simulink model "UnderwaterGliderLongModel2021b"  (R2021b)
settings: Solver=VariableStepAuto  StartTime=0.0  StopTime=inf  FixedStep=0.0000111111111111111111111111111  RelTol=1e-3
values from neighbouring files (symbols this model uses):
  mb = 1.0    (= 1)    [Initialization.m]
  mb_d = (m - mbar - mh - ms -mw) + (1/g)*( (-sin(xi_d))*(KD0 + KD*(alpha_d^2)) + (cos(xi_d))*(KL0 + KL*(alpha_d)))*(V_d^2)    [Initialization.m]
  rb1 = 0.00    (= 0)    [Initialization.m]
  rb3 = 0.00    (= 0)    [Initialization.m]
  rp1_d = (1/(mbar + lambda*ms))*(-mb_d*rb1 -tan(theta_d)*(mbar*rp3 + ms*rs3 + mb*rb3) + (1/(g*cos(theta_d)))*((mf3 - mf1)*v1_d*v3_d + (KM0 + KM*alpha_d)*(V_d^2)))    [Initialization.m]
  rp3 = 0.05    [Initialization.m]
  rs1_d = lambda*rp1_d    [Initialization.m]
  rs3 = 0.00    (= 0)    [Initialization.m]
  theta0 = 0.4    [Initialization.m]
  v1_d = V_d*cos(alpha_d)    [Initialization.m]
  v3_d = V_d*sin(alpha_d)    [Initialization.m]
libraries: aerolibfltsims x2, aerolibanim x1
settings Model: Creator=AAAR  LastModifiedBy=AAAR
settings DebuggingCC: UnconnectedInputMsg=none  UnconnectedOutputMsg=none  UnconnectedLineMsg=none
settings ModelReferenceCC: EnableRefExpFcnMdlSchedulingChecks=off
settings RTWCC: GPUComputeCapability=5.0  DLArmComputeVersion=20.02.1

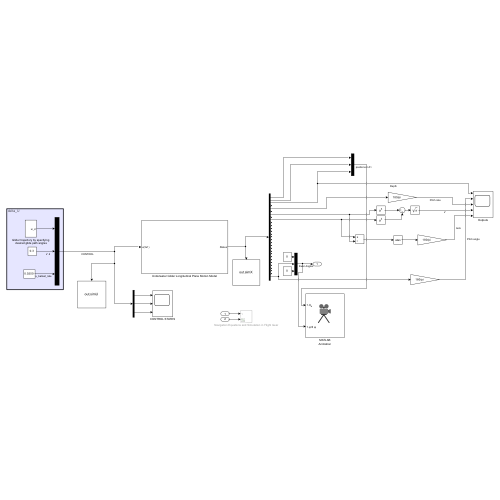
[thumbnail: Simulink's stored preview of the top-level diagram]
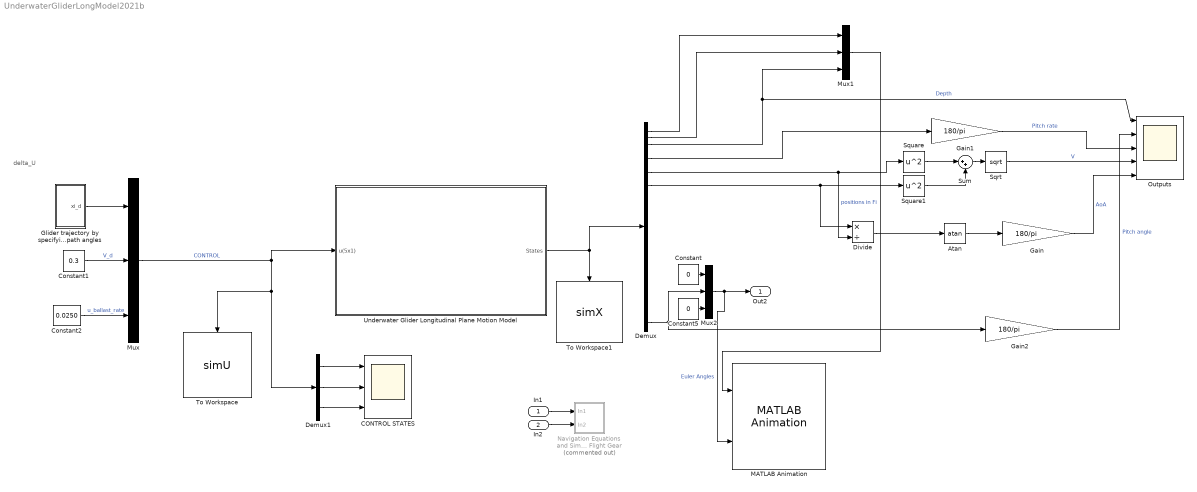
== system UnderwaterGliderLongModel2021b ==
  note: delta_U
  In1 : Inport
  In2 : Inport  Port=2
  Atan : Trigonometry  Operator=atan
  "CONTROL STATES " : Scope  NumInputPorts=3
  Constant : Constant  Value=0
  Constant1 : Constant  Value=0.3
  Constant2 : Constant  Value=0.0250
  Constant5 : Constant  Value=0
  Demux : Demux  Outputs=29
  Demux1 : Demux  Outputs=3
  Divide : Product  Inputs=*/
  Gain : Gain  Gain=180/pi
  Gain1 : Gain  Gain=180/pi
  Gain2 : Gain  Gain=180/pi
  Glider trajectory by specifying desired glide path angles : Subsystem
  MATLAB Animation : aerolibanim/MATLAB Animation  Tag=Matlab Animation 6 DOF  Vehicles=1  Geometries='pa24-250_orange.ac'  BoundingBoxCoordinates=[-50,50,-50,50,-50,50]  CameraOffset=[-150,-50,0]  CameraViewAngle=3  SampleTime=0.2  FigurePosition=[636,187,619,597]
  Mux : Mux  Inputs=3
  Mux1 : Mux  Inputs=3
  Mux2 : Mux  Inputs=3
  Navigation Equations and Simulation in Flight Gear : Subsystem  Commented=on
  Outputs : Scope  NumInputPorts=5
  Sqrt : Sqrt  SaturateOnIntegerOverflow=on
  Square : Math  Operator=square  SaturateOnIntegerOverflow=on
  Square1 : Math  Operator=square  SaturateOnIntegerOverflow=on
  Sum : Sum  Inputs=|++
  To Workspace : ToWorkspace  VariableName=simU  SaveFormat=Timeseries  SampleTime=-1
  To Workspace1 : ToWorkspace  VariableName=simX  SaveFormat=Timeseries  SampleTime=-1
  Underwater Glider Longitudinal Plane Motion Model : Subsystem
  Out2 : Outport
  wires:
  Mux/1 -> Underwater Glider Longitudinal Plane Motion Model/1(u(5x1)), Demux1/1, To Workspace/1  "CONTROL"
  Underwater Glider Longitudinal Plane Motion Model/1(States) -> Demux/1, To Workspace1/1
  Mux2/1 -> MATLAB Animation/2, Out2/1  "Euler Angles"
  Constant1/1 -> Mux/2  "V_d"
  Constant2/1 -> Mux/3  "u_ballast_rate"
  In1/1 -> Navigation Equations and Simulation in Flight Gear/1(In1)
  In2/1 -> Navigation Equations and Simulation in Flight Gear/2(In2)
  Glider trajectory by specifying desired glide path angles/1(xi_d) -> Mux/1
  Constant/1 -> Mux2/1
  Constant5/1 -> Mux2/3
  Demux/29 -> Gain2/1, Mux2/2
  Demux/1 -> Mux1/1
  Demux/2 -> Mux1/2
  Demux/3 -> Outputs/1, Mux1/3  "Depth"
  Mux1/1 -> MATLAB Animation/1  "positions in Fi"
  Demux/5 -> Gain1/1
  Demux/7 -> Square/1, Divide/2
  Square/1 -> Sum/1
  Square1/1 -> Sum/2
  Sum/1 -> Sqrt/1
  Sqrt/1 -> Outputs/4  "V"
  Divide/1 -> Atan/1
  Atan/1 -> Gain/1
  Gain/1 -> Outputs/5  "AoA"
  Demux1/1 -> "CONTROL STATES "/1
  Demux1/2 -> "CONTROL STATES "/2
  Demux1/3 -> "CONTROL STATES "/3
  Gain1/1 -> Outputs/3  "Pitch rate"
  Demux/9 -> Divide/1, Square1/1
  Gain2/1 -> Outputs/2  "Pitch angle"

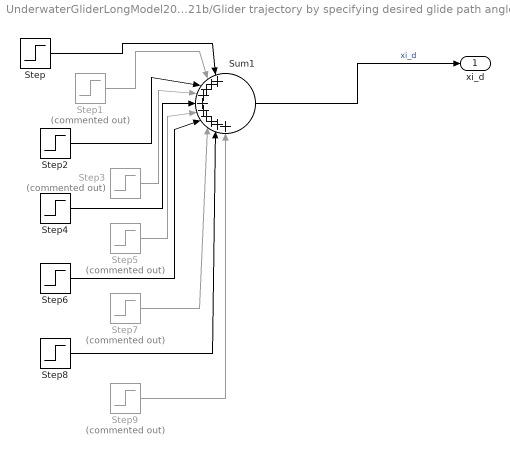
== system UnderwaterGliderLongModel2021b/Glider trajectory by specifying desired glide path angles ==
  Step : Step  Time=0  After=-25*(pi/180)  SampleTime=0
  Step1 : Step  Commented=on  Time=15+5  After=25*(pi/180)  SampleTime=0
  Step2 : Step  Time=375  After=50*(pi/180)  SampleTime=0
  Step3 : Step  Commented=on  Time=50+5  After=-25*(pi/180)  SampleTime=0
  Step4 : Step  Time=750  After=-50*(pi/180)  SampleTime=0
  Step5 : Step  Commented=on  Time=80+5  After=25*(pi/180)  SampleTime=0
  Step6 : Step  Time=1125  After=50*(pi/180)  SampleTime=0
  Step7 : Step  Commented=on  Time=110+5  After=-25*(pi/180)  SampleTime=0
  Step8 : Step  Time=1500  After=-50*(pi/180)  SampleTime=0
  Step9 : Step  Commented=on  Time=130+5  After=25*(pi/180)  SampleTime=0
  Sum1 : Sum  Inputs=|++++++++++
  xi_d : Outport
  wires:
  Step5/1 -> Sum1/6
  Step/1 -> Sum1/1
  Step8/1 -> Sum1/9
  Step3/1 -> Sum1/4
  Step1/1 -> Sum1/2
  Step6/1 -> Sum1/7
  Step9/1 -> Sum1/10
  Step2/1 -> Sum1/3
  Step4/1 -> Sum1/5
  Step7/1 -> Sum1/8
  Sum1/1 -> xi_d/1  "xi_d"

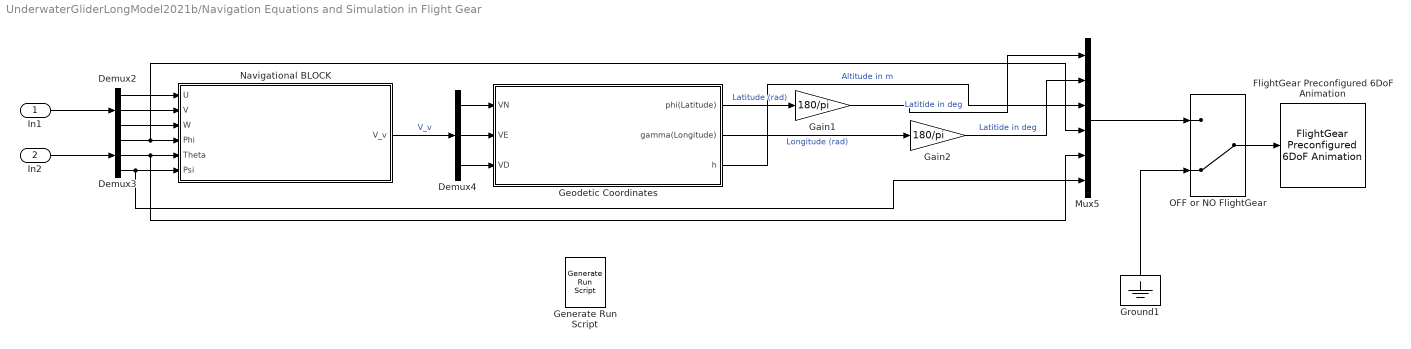
== system UnderwaterGliderLongModel2021b/Navigation Equations and Simulation in Flight Gear ==
  In1 : Inport
  In2 : Inport  Port=2
  Demux2 : Demux  Outputs=3
  Demux3 : Demux  Outputs=3
  Demux4 : Demux  Outputs=3
  FlightGear Preconfigured 6DoF Animation : aerolibfltsims/FlightGear Preconfigured 6DoF Animation  xFlightGearVersion=v2019.1  DestinationIpAddress=127.0.0.1  DestinationPort=5502  SampleTime=1/30  packetVersion=24
  Gain1 : Gain  Gain=180/pi
  Gain2 : Gain  Gain=180/pi
  Generate Run Script : aerolibfltsims/Generate Run Script  Architecture=Win64  dataFlow=Send  GeometryModelName=c172p  AirportId=KSFO  RunwayId=10L  InitialAltitude=7224  InitialHeading=113  OffsetDistance=4.72  OffsetAzimuth=0  InstallScenery=off  DisableShaders=off  OriginAddress=127.0.0.1  DestinationPort=5502  OriginPort=5505  LocalAddress=127.0.0.1  OutputFileName=runfg.bat  FlightGearBaseDirectory=E:\$ 00 My Data\FlightGear 2020.3
  Geodetic Coordinates : Subsystem
  Ground1 : Ground
  Mux5 : Mux  Inputs=6
  Navigational BLOCK : Subsystem
  OFF or NO FlightGear : ManualSwitch  CurrentSetting=0
  wires:
  Demux2/3 -> Navigational BLOCK/3(W)
  Demux4/2 -> Geodetic Coordinates/2(VE)
  Gain2/1 -> Mux5/2  "Latitide in deg"
  Geodetic Coordinates/1(phi(Latitude)) -> Gain1/1  "Latitude (rad)"
  Demux3/1 -> Mux5/4, Navigational BLOCK/4(Phi)
  Demux2/1 -> Navigational BLOCK/1(U)
  Demux2/2 -> Navigational BLOCK/2(V)
  Ground1/1 -> OFF or NO FlightGear/2
  Demux3/2 -> Mux5/5, Navigational BLOCK/5(Theta)
  Demux4/3 -> Geodetic Coordinates/3(VD)
  In1/1 -> Demux2/1
  Geodetic Coordinates/3(h) -> Mux5/3  "Altitude in m"
  OFF or NO FlightGear/1 -> FlightGear Preconfigured 6DoF Animation/1
  Demux4/1 -> Geodetic Coordinates/1(VN)
  Navigational BLOCK/1(V_v) -> Demux4/1  "V_v"
  Geodetic Coordinates/2(gamma(Longitude)) -> Gain2/1  "Longitude (rad)"
  In2/1 -> Demux3/1
  Gain1/1 -> Mux5/1  "Latitide in deg"
  Demux3/3 -> Mux5/6, Navigational BLOCK/6(Psi)
  Mux5/1 -> OFF or NO FlightGear/1

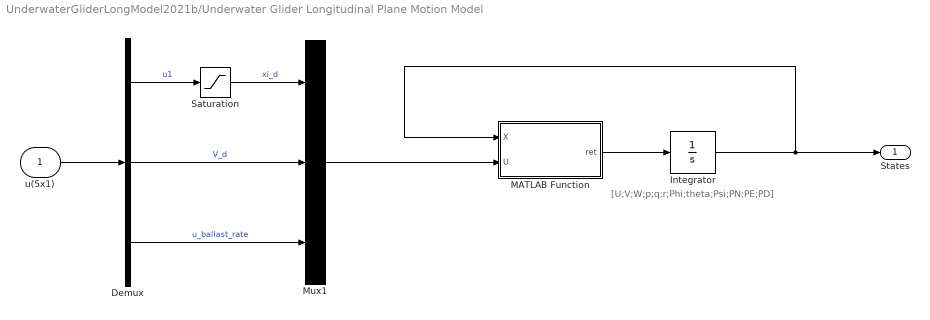
== system UnderwaterGliderLongModel2021b/Underwater Glider Longitudinal Plane Motion Model ==
  note: [U;V;W;p;q;r;Phi;theta;Psi;PN;PE;PD]
  u(5x1) : Inport
  Demux : Demux  Outputs=3
  Integrator : Integrator  InitialCondition=[0; 0; 0; 0; 0; 0; v1_d; 0; v3_d; rp1_d; 0; rp3; rs1_d; 0; rs3; rb1; 0; rb3; 0; 0; 0; 0; 0; 0; mb*v1_d; 0; mb*v3_d; mb_d; theta0]
  MATLAB Function : MATLAB Function  TreatAsAtomicUnit=on
  Mux1 : Mux  Inputs=3
  Saturation : Saturate  UpperLimit=6.314842  LowerLimit=-6.314842
  States : Outport
  wires:
  Demux/2 -> Mux1/2  "V_d"
  Demux/3 -> Mux1/3  "u_ballast_rate"
  MATLAB Function/1(ret) -> Integrator/1
  Integrator/1 -> MATLAB Function/1(X), States/1
  Demux/1 -> Saturation/1  "u1"
  Saturation/1 -> Mux1/1  "xi_d"
  Mux1/1 -> MATLAB Function/2(U)
  u(5x1)/1 -> Demux/1

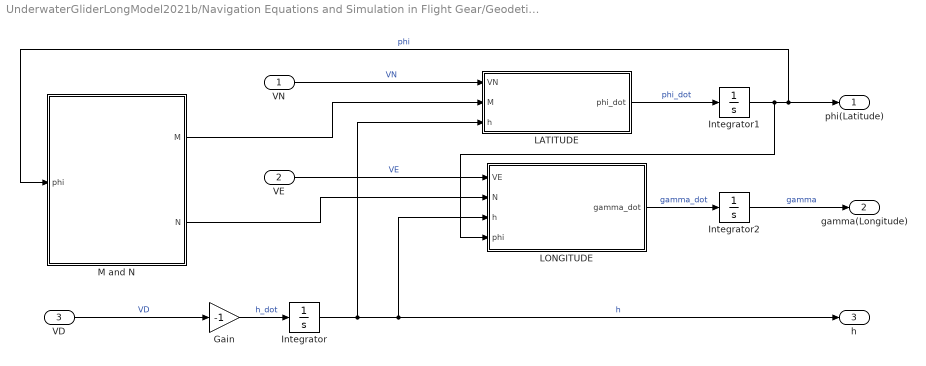
== system UnderwaterGliderLongModel2021b/Navigation Equations and Simulation in Flight Gear/Geodetic Coordinates ==
  VN : Inport
  VE : Inport  Port=2
  VD : Inport  Port=3
  Gain : Gain  Gain=-1
  Integrator : Integrator  InitialCondition=150
  Integrator1 : Integrator  InitialCondition=0.22181
  Integrator2 : Integrator  InitialCondition=1.356068
  LATITUDE : MATLAB Function  TreatAsAtomicUnit=on
  LONGITUDE : MATLAB Function  TreatAsAtomicUnit=on
  M and N : Subsystem
  phi(Latitude) : Outport
  gamma(Longitude) : Outport  Port=2
  h : Outport  Port=3
  wires:
  VD/1 -> Gain/1  "VD"
  Gain/1 -> Integrator/1  "h_dot"
  Integrator/1 -> LATITUDE/3(h), LONGITUDE/3(h), h/1  "h"
  M and N/1(M) -> LATITUDE/2(M)
  M and N/2(N) -> LONGITUDE/2(N)
  LATITUDE/1(phi_dot) -> Integrator1/1  "phi_dot"
  Integrator1/1 -> LONGITUDE/4(phi), M and N/1(phi), phi(Latitude)/1  "phi"
  VE/1 -> LONGITUDE/1(VE)  "VE"
  VN/1 -> LATITUDE/1(VN)  "VN"
  LONGITUDE/1(gamma_dot) -> Integrator2/1  "gamma_dot"
  Integrator2/1 -> gamma(Longitude)/1  "gamma"

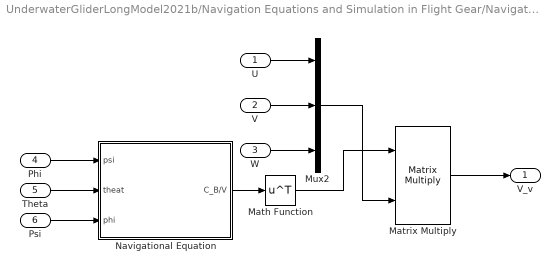
== system UnderwaterGliderLongModel2021b/Navigation Equations and Simulation in Flight Gear/Navigational BLOCK ==
  U : Inport
  V : Inport  Port=2
  W : Inport  Port=3
  Phi : Inport  Port=4
  Theta : Inport  Port=5
  Psi : Inport  Port=6
  Math Function : Math  Operator=transpose  SaturateOnIntegerOverflow=on
  Matrix Multiply : Product  Multiplication=Matrix(*)
  Mux2 : Mux  Inputs=3
  Navigational Equation : Subsystem
  V_v : Outport
  wires:
  Mux2/1 -> Matrix Multiply/2
  Math Function/1 -> Matrix Multiply/1
  Phi/1 -> Navigational Equation/1(psi)
  U/1 -> Mux2/1
  Theta/1 -> Navigational Equation/2(theat)
  Matrix Multiply/1 -> V_v/1
  Navigational Equation/1(C_B/V) -> Math Function/1
  W/1 -> Mux2/3
  Psi/1 -> Navigational Equation/3(phi)
  V/1 -> Mux2/2

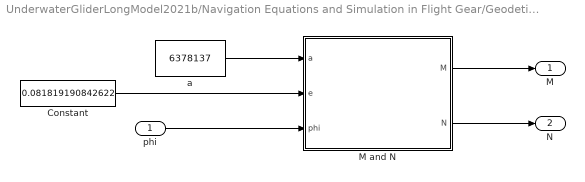
== system UnderwaterGliderLongModel2021b/Navigation Equations and Simulation in Flight Gear/Geodetic Coordinates/M and N ==
  phi : Inport
  Constant : Constant  Value=0.081819190842622
  M and N : MATLAB Function  TreatAsAtomicUnit=on
  a : Constant  Value=6378137
  M : Outport
  N : Outport  Port=2
  wires:
  Constant/1 -> M and N/2(e)
  phi/1 -> M and N/3(phi)
  M and N/1(M) -> M/1
  a/1 -> M and N/1(a)
  M and N/2(N) -> N/1

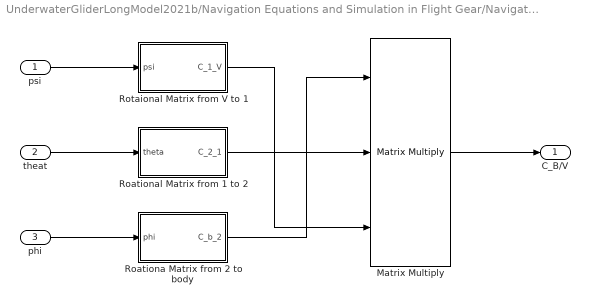
== system UnderwaterGliderLongModel2021b/Navigation Equations and Simulation in Flight Gear/Navigational BLOCK/Navigational Equation ==
  psi : Inport
  theat : Inport  Port=2
  phi : Inport  Port=3
  Matrix Multiply : Product  Inputs=3  Multiplication=Matrix(*)
  Roationa Matrix from 2 to body : MATLAB Function  TreatAsAtomicUnit=on
  Roational Matrix from 1 to 2 : MATLAB Function  TreatAsAtomicUnit=on
  Rotaional Matrix from V to 1 : MATLAB Function  TreatAsAtomicUnit=on
  C_B/V : Outport
  wires:
  Matrix Multiply/1 -> C_B/V/1
  Rotaional Matrix from V to 1/1(C_1_V) -> Matrix Multiply/3
  Roational Matrix from 1 to 2/1(C_2_1) -> Matrix Multiply/2
  Roationa Matrix from 2 to body/1(C_b_2) -> Matrix Multiply/1
  phi/1 -> Roationa Matrix from 2 to body/1(phi)
  theat/1 -> Roational Matrix from 1 to 2/1(theta)
  psi/1 -> Rotaional Matrix from V to 1/1(psi)

== matlab function UnderwaterGliderLongModel2021b/Navigation Equations and Simulation in Flight Gear/Navigational BLOCK/Navigational Equation/Roational Matrix from 1 to 2 ==
  data: theta input; C_2_1 output
function C_2_1 = fcn(theta)

% Roational Matrix From the 1 frame to 2 frame

C_2_1=[cos(theta) 0 -sin(theta); 0 1 0; sin(theta) 0 cos(theta)];

end

== matlab function UnderwaterGliderLongModel2021b/Underwater Glider Longitudinal Plane Motion Model/MATLAB Function ==
  data: X input; U input; ret output
function ret=Model3d(X, U)

%% Define terms

b       = X(1:3);                 % Position in earth frame
Omega   = X(4:6);                 % Angular rate
v       = X(7:9);                 % Velocity in body frame
rp      = X(10:12);               % Position of primary moving mass
rs      = X(13:15);               % Position of secondary moving mass
rb      = X(16:18);               % Position of ballast mass
Pp      = X(19:21);               % Linear momentum of primary moving mass
Ps      = X(22:24);               % Linear momentum of secondary moving mass
Pb      = X(25:27);               % Linear momentum of ballast moving mass
mb      = X(28);                  % Ballast mass
theta   = X(29);                  % Pitch
alpha = atan(v(3)/v(1));          % Angle of attack

%% Constants

g = 9.816;                  % Acceleration due to gravity
I3 = eye(3);                % Identity matrix (3x3)
Z3 = zeros(3);              % Zero matrix (3x3)

i = [1 0 0]';               % Unit vector along earth frame x-axis
j = [0 1 0]';               % Unit vector along earth frame y-axis
k = [0 0 1]';               % Unit vector along earth frame z-axis

%% Mass Properties

mh = 40;                        % Hull mass
mbar = 9;                       % Primary moving inernal mass
ms = 0;                         % Secondary moving inernal mass
mb = 1.0;                       % Variable ballast mass     
mw = 0;                         % Fixed point mass
mv = mh + mw + ms + mb + mbar;  % Total vehicle mass
m = 50;                         % Displacement
m0 = mv - m;                    % Buoyancy

mf1 = 5;                        % Added mass term
mf2 = 60;                       % Added mass term
mf3 = 70;                       % Added mass term     
Mf = diag([mf1, mf2, mf3]);     % Added mass matrix

M = mh*I3 + Mf;                 % Total mass
Minv = inv(M);
m1 = M(1,1);    
m2 = M(2,2);
m3 = M(3,3);

j1 = 4;                         % Inertia term  
j2 = 12;                        % Inertia term
j3 = 11;                        % Inertia term
J = diag([j1, j2, j3]);         % Total inertia
Jinv = inv(J);

%% Force and Moment Coefficients 

KL = 132.5;                 % Lift coefficient
KL0 = 0;                    % Lift coefficient

KD = 25;                    % Drag Coefficient
KD0 = 2.15;                 % Drag Coefficient

KM = -100;                  % Moment Coefficient
KM0 = 0;                    % Moment Coefficient

KOmega1_2 = -50;            % Rotational Damping Coefficient
KOmega2_2 = -50;            % Rotational Damping Coefficient

%% Set glider inputs (constant states)

rp3 = 0.05;                 % Fixed position of primary moving mass in body coordinate along e3 axis
rs3 = 0.00;                 % Fixed position of secondary moving mass in body coordinate along e3 axis
rb1 = 0.00;                 % Fixed position of ballast mass in body coordinate along e1 axis
rb3 = 0.00;                 % Fixed position of ballast mass in body coordinate along e3 axis
phi = 0;                    % Glider roll angle
yaw = 0;                    % Glider yaw angle

%% Control inputs and their desired state values

xi_d           = U(1);                   % Desired flight path angle
V_d            = U(2);                   % Desired vertical speed in earth frame
u_ballast_rate = U(3);                   % Ballast rate input (kg/s) (Magnitude only, sign is assigned later - by the model)

% Get glide direction & ballast rate from input glide path angle
    % Glide direction (1 = Upwards, -1 = Downwards)
glide_dir = -1;           % Initial value to avoid error in code generation in simulink
    if xi_d > 0
        glide_dir = 1;
        u_ballast_rate = -abs(u_ballast_rate);          % Negative ballast rate for upward glide
    elseif xi_d < 0
        glide_dir = -1;
        u_ballast_rate = abs(u_ballast_rate);           % Positive ballast rate for downward glide
    end

% Desired state values calculations
% Desired angle of attack
% if (1 - 4*(KD/(KL^2))*(cot(xi_d))*(KD0*cot(xi_d) + KL0) < 0) alpha_d=0; else % Error handling
alpha_d = (1/2)*(KL/KD)*(tan(xi_d))*(-1 + sqrt(1 - 4*(KD/(KL^2))*(cot(xi_d))*(KD0*cot(xi_d) + KL0))); % end
% Desired velocity in body frame
v1_d = V_d*cos(alpha_d);
v3_d = V_d*sin(alpha_d);
% Desired ballast mass
mb_d = (m - mbar - mh - ms -mw) + (1/g)*( (-sin(xi_d))*(KD0 + KD*(alpha_d^2)) + (cos(xi_d))*(KL0 + KL*(alpha_d)))*(V_d^2);
% Desired position of longitudinal moving masses
lambda = 1;
theta_d = alpha_d + xi_d;

rp1_d = (1/(mbar + lambda*ms))*(-mb_d*rb1 -tan(theta_d)*(mbar*rp3 + ms*rs3 + mb*rb3) + (1/(g*cos(theta_d)))*((mf3 - mf1)*v1_d*v3_d + (KM0 + KM*alpha_d)*(V_d^2)));
rs1_d = lambda*rp1_d;


%% Check on ballast mass

if glide_dir == 1
    if mb <= mb_d
        mb = mb_d;              % Turn off ballast when desired mass is obtained
    end    
elseif glide_dir == -1
    if mb >= mb_d
        mb = mb_d;              % Turn off ballast when desired mass is obtained
    end  
end
 
%% Position Vectors

% Limit the longitudinal position of moving masses
if glide_dir == 1               % During upward glide primary moving mass moves in negative e1 direction
    if rp(1) <= rp1_d
        rp(1) = rp1_d;
    end
    if rs(1) <= rs1_d
        rs(1) = rs1_d;
    end
elseif glide_dir == -1          % During downward glide primary moving mass moves in positive e1 direction
    if rp(1) >= rp1_d
        rp(1) = rp1_d;
    end 
    if rs(1) >= rs1_d
        rs(1) = rs1_d;
    end 
end

% Primary moving mass
rp_c = [ 0      -rp(3)  rp(2)
         rp(3)  0       -rp(1)
        -rp(2)  rp(1)   0  ];
    
% Secondary moving mass
rs_c = [ 0      -rs(3)  rs(2)
         rs(3)  0       -rs(1)
        -rs(2)  rs(1)   0  ];

% Ballast mass
rb_c = [ 0      -rb(3)  rb(2)
         rb(3)  0       -rb(1)
        -rb(2)  rb(1)   0  ]; 
    
    
%% Transformation matrix

R = [cos(yaw)*cos(theta)    (-sin(yaw)*cos(phi) + cos(yaw)*sin(theta)*sin(phi)) (sin(yaw)*sin(phi) + cos(yaw)*cos(phi)*sin(theta))
     sin(yaw)*cos(theta)    (cos(yaw)*cos(phi) + sin(phi)*sin(theta)*sin(yaw))  (-cos(yaw)*sin(phi) + sin(theta)*sin(yaw)*cos(phi))
     -sin(theta)            cos(theta)*sin(phi)                                 cos(theta)*cos(phi)];

RT = R';

%% Force and Torque terms

L = (KL0 + KL*((alpha)))*(v(1)^2 + v(3)^2);                      % Lift force                         
D = (KD0 + KD*((alpha))^2)*(v(1)^2 + v(3)^2);                    % Drag force
MDL = (KM0 + KM*((alpha)))*(v(1)^2 + v(3)^2) ...                 % Moment
      + KOmega1_2*Omega(2) + KOmega2_2*(Omega(2)^2);

F_ext = [-D 0 -L]';                                          % Total external force
T_ext = [0 MDL 0]';                                          % Total external mmoment

%% Internal Mass Velocity Vectors

% Limit the rate of movement of primary moving mass
rp_dot = [0 0 0]';      % Initial value to avoid error in code generation in simulink
rs_dot = [0 0 0]';      % Initial value to avoid error in code generation in simulink
if glide_dir == 1
    rp_dot = (1/mbar)*Pp - v - cross(Omega, rp);             % rp_dot in upward glide
    if ms > 0                                                
       rs_dot = (1/ms)*Ps - v - cross(Omega, rs);            % rs_dot in upward glide
    else
       rs_dot = [0 0 0]'; 
    end
    
    if rp(1) <= rp1_d                                        % When desired value reached, set rate = 0
        rp_dot = [0 0 0]';
    end
    if rs(1) <= rs1_d                                        % When desired value reached, set rate = 0
        rs_dot = [0 0 0]';
    end
elseif glide_dir == -1
    rp_dot = (1/mbar)*Pp + v - cross(Omega, rp);             % rp_dot in upward glide
    if ms > 0                                                
       rs_dot = (1/ms)*Ps + v - cross(Omega, rs);            % rs_dot in upward glide
    else
       rs_dot = [0 0 0]'; 
    end
    
    if rp(1) >= rp1_d                                        % When desired value reached, set rate = 0
        rp_dot = [0 0 0]';
    end
    if rs(1) >= rs1_d                                        % When desired value reached, set rate = 0
        rs_dot = [0 0 0]';
    end
end

rb_dot = [0 0 0]';                                           % rb_dot

%% Momentum Matrix

Pb = mb*(v + cross(Omega,rb) + rb_dot);                     % Linear momentum of ballast mass

%% Calculate net buoyancy

m0 = mh + mw + mb + ms + mbar - m;

%% Control Inputs

% Set acceleration input of primary moving mass
wp1 = 0.02;           % Initial value to avoid error in code generation in simulink
if glide_dir == 1
    wp1 = -0.02;            % wp1 in upward glide (m/s^2)
elseif glide_dir == -1 
    wp1 = 0.02;             % wp1 in downward glide (m/s^2)
end
wp2 = 0;                    % wp2
wp3 = 0;                    % wp3

wp = [wp1                   % (w1) Accleration input of movable point mass mbar along body axis e1
      wp2                   % (w2) Accleration input of movable point mass mbar along body axis e2
      wp3];                 % (w3) Accleration input of movable point mass mbar along body axis e3

% Accleration input of ballast point mass mb in body coordinates
wb = 0;  
 
% Check on ballast rate
if glide_dir == 1
    if mb <= mb_d
        u_ballast_rate = 0;             % Turn off ballast when desired mass is obtained
    end    
elseif glide_dir == -1
    if mb >= mb_d
        u_ballast_rate = 0;             % Turn off ballast when desired mass is obtained
    end  
end

%% Control Transformation

F = [ (Minv - rp_c*Jinv*rp_c + (I3/mbar))       (Minv - rp_c*Jinv*rb_c)               
      (Minv - rb_c*Jinv*rp_c)                   (Minv - rb_c*Jinv*rb_c + (I3/mb))];    

H = inv(F);

Zp = -Minv*[cross((M*v + Pp + Pb),Omega) + m0*g*RT*k + F_ext] - cross(Omega,rp_dot) ...
      -Jinv*cross([cross((J*Omega + rp_c*Pp + rb_c*Pb),Omega) + cross((M*v),v) + T_ext ...
      + cross(cross(Omega,rp),Pp) + cross(cross(Omega,rb),Pb) ...
      + (mbar*rp_c + mb*rb_c)*g*RT*k],rp);

Zb = -Minv*[cross((M*v + Pp + Pb),Omega) + m0*g*RT*k + F_ext] - cross(Omega,rb_dot) ...
     -Jinv*cross([cross((J*Omega + rp_c*Pp + rb_c*Pb),Omega) + cross((M*v),v) + T_ext ...
     + cross(cross(Omega,rp),Pp) + cross(cross(Omega,rb),Pb) ...
     + (mbar*rp_c + mb*rb_c)*g*RT*k],rb);
  
 u = H*[(-Zp + wp)
        (-Zb + wb)];
    
 %% Control Inputs
 
 u_bar = [0 0 0]';               % Initial value to avoid error in code generation in simulink
 us    = [0 0 0]';               % Initial value to avoid error in code generation in simulink
 if glide_dir == 1
     
    if rp(1) <= rp1_d
        u_bar = [0 0 0]';
    else
        u_bar = [-0.18 0 0]';
        %u_bar = [u(1) 0 0]';
    end 
    
    if rs(1) <= rs1_d
        us    = [0 0 0]';
    else
        us    = [-0.18 0 0]';
    end
     
    if ms == 0                              % If secondary mass doed not exist
        us    = [0 0 0]';
    end
    
 elseif glide_dir == -1
    
    if rp(1) >= rp1_d
        u_bar = [0 0 0]';
    else
        u_bar = [0.18 0 0]';
        %u_bar = [u(1) 0 0]';
    end 
    
    if rs(1) >= rs1_d
        us    = [0 0 0]';
    else
        us    = [0.18 0 0]';
    end
    
    if ms == 0                              % If secondary mass doed not exist
        us    = [0 0 0]';
    end
 end
 
 ub = [0 0 0]';

%% Equations of motion

T_bar      = cross((J*Omega + rp_c*Pp + rs_c*Ps + rb_c*Pb), Omega) + cross((M*v),v) ...
             + cross(cross(Omega, rp), Pp) + + cross(cross(Omega, rs), Ps) + + cross(cross(Omega, rb), Pb) + (mbar*rp_c + ms*rs_c + mb*rb_c)*g*RT*k ...
             + T_ext - rp_c*u_bar - rs_c*us - rb_c*ub;

F_bar      = cross((M*v + Pp + Ps + Pb), Omega) + m0*g*RT*k + F_ext - u_bar - us - ub;

b_dot      = R*v;
Omega_dot  = Jinv*T_bar;
v_dot      = Minv*F_bar;
% rp_dot     = (1/mbar)*Pp - v - cross(Omega, rp);
% rs_dot     = (1/ms)*Pd - v - cross(Omega, rs);
% rb_dot     = (1/mb)*Pb - v - cross(Omega, rb);
Pp_dot     = u_bar;
Ps_dot     = us;
Pb_dot     = ub;
mb_dot     = u_ballast_rate;
theta_dot  = Omega(2);

%% Return

ret = [b_dot' Omega_dot' v_dot' rp_dot' rs_dot' rb_dot' Pp_dot' Ps_dot' Pb_dot' mb_dot theta_dot]';

== matlab function UnderwaterGliderLongModel2021b/Navigation Equations and Simulation in Flight Gear/Navigational BLOCK/Navigational Equation/Roationa Matrix from 2 to body ==
  data: phi input; C_b_2 output
function C_b_2 = fcn(phi)

% Roational Matrix from the 2 frame to body frame
C_b_2=[1 0 0; 0 cos(phi) sin(phi); 0 -sin(phi) cos(phi)];
end

== matlab function UnderwaterGliderLongModel2021b/Navigation Equations and Simulation in Flight Gear/Navigational BLOCK/Navigational Equation/Rotaional Matrix from V to 1 ==
  data: psi input; C_1_V output
function C_1_V = fcn(psi)

% Calculating the Rotaional Matrix  from the NED to 1 frame

C_1_V=[cos(psi) sin(psi) 0; -sin(psi) cos(psi) 0; 0 0 1];

end

== matlab function UnderwaterGliderLongModel2021b/Navigation Equations and Simulation in Flight Gear/Geodetic Coordinates/LATITUDE ==
  data: VN input; phi_dot output; M input; h input
function phi_dot =Latitude_Rate(VN,M,h)
% Calculating the Rate of change of Latitude

phi_dot=VN/(M+h);
end

== matlab function UnderwaterGliderLongModel2021b/Navigation Equations and Simulation in Flight Gear/Geodetic Coordinates/LONGITUDE ==
  data: VE input; gamma_dot output; N input; h input; phi input
function gamma_dot =Longitude_Rate(VE,N,h,phi)

% Calculating the Rate of change of the Longitude

gamma_dot=VE/((N+h)*cos(phi));
end

== matlab function UnderwaterGliderLongModel2021b/Navigation Equations and Simulation in Flight Gear/Geodetic Coordinates/M and N/M and N ==
  data: a input; M output; e input; phi input; N output
function[M,N]=M_N(a,e,phi)

M=(a*(1-e*2)/(1-(e^2)*sin(phi))^3/2);  % Meridian Radius of Curvature

N=a/(1-(e^2)*(sin(phi)^2))^3/2;        % Prime verical radius of curvature

end
